simulink model "modelsim_single"  (R2016a)
settings: Solver=ode4  StartTime=0.0  StopTime=Tfinal  FixedStep=Ts  RelTol=1e-3
values from neighbouring files (symbols this model uses):
  Cdc = 100e-6    (= 0.0001)    [codemodel.m]
  delta = acos(Efm/Vt)    [codemodel.m]
  deltad = delta*180/pi    [codemodel.m]
  Ef = 155    [codemodel.m]
  fout = 50    [codemodel.m]
  Ls = 13.8e-3    (= 0.0138)    [codemodel.m]
  ma = Vt*sqrt(3)/(Vdcm*0.612)    [codemodel.m]
  phase = [0 0]    [codemodel.m]
  Rin = 10    [codemodel.m]
  Ripth = 0.08    [codemodel.m]
  Rs = 1e-9    (= 1e-09)    [codemodel.m]
  Ts = 1e-6    (= 1e-06)    [codemodel.m]
  Vin = Vdc + Rin*(Pout/Vdc)    (= 697.604412924)    [codemodel.m]
  wout = 2*pi*fout    (= 314.159265359)    [codemodel.m]
undefined symbols (not defined in the file or in its folder): Lload, Rload
libraries: powerlib x28, powerlib_meascontrol x13, simulink x2
settings Model: Creator=ugurm  LastModifiedBy=mesutto
settings DataIOCC: LimitDataPoints=on  SaveFormat=Array
settings DebuggingCC: UnderspecifiedInitializationDetection=Classic  MergeDetectMultiDrivingBlocksExec=none  SolverPrmCheckMsg=warning  StateNameClashWarn=warning
settings HardwareCC: ProdBitPerPointer=32  ProdLargestAtomicFloat=None  ProdIntDivRoundTo=Undefined  ProdEndianess=Unspecified  ProdWordSize=32  ProdHWDeviceType=32-bit Generic
settings ModelReferenceCC: PropagateSignalLabelsOutOfModel=off
settings ConfigComp: CovModelRefEnable=Off

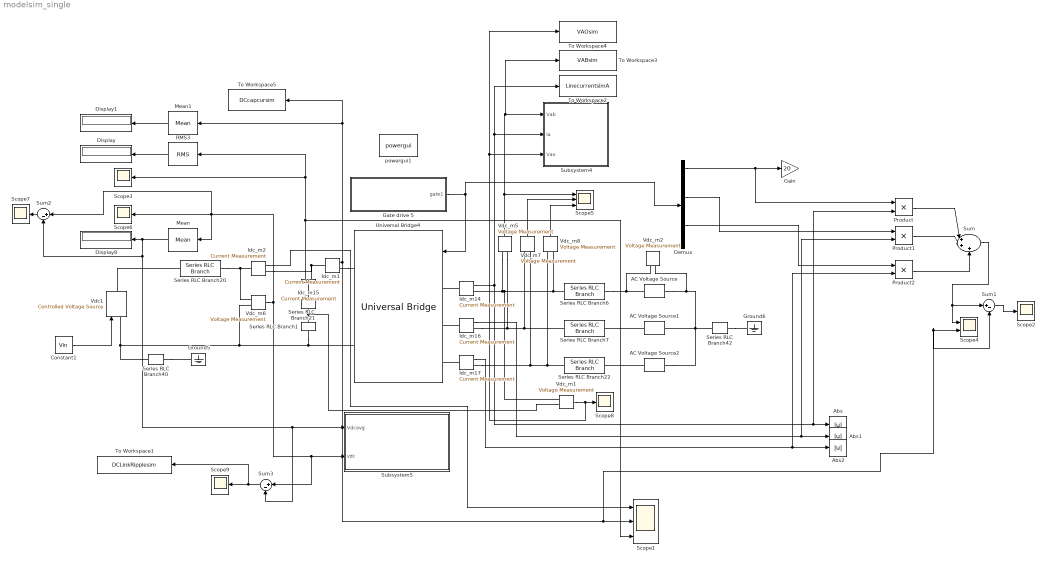
== system modelsim_single ==
  AC Voltage Source : powerlib/Electrical Sources/AC Voltage Source  Amplitude=Ef*sqrt(2)  Phase=0  Frequency=fout  SampleTime=0  Measurements=None  BusType=swing  Pref=10e3  Qref=0  Qmin=-inf  Qmax=+inf
  AC Voltage Source1 : powerlib/Electrical Sources/AC Voltage Source  Amplitude=Ef*sqrt(2)  Phase=-120  Frequency=fout  SampleTime=0  Measurements=None  BusType=swing  Pref=10e3  Qref=0  Qmin=-inf  Qmax=+inf
  AC Voltage Source2 : powerlib/Electrical Sources/AC Voltage Source  Amplitude=Ef*sqrt(2)  Phase=-240  Frequency=fout  SampleTime=0  Measurements=None  BusType=swing  Pref=10e3  Qref=0  Qmin=-inf  Qmax=+inf
  Abs : Abs
  Abs1 : Abs
  Abs2 : Abs
  Constant1 : Constant  Value=Vin
  Demux : Demux  Outputs=6
  Display : Display
  Display1 : Display
  Display8 : Display
  Gain : Gain  Gain=20
  Gate drive 5 : Subsystem
  Ground5 : powerlib/Elements/Ground  LConnTagsString=a
  Ground6 : powerlib/Elements/Ground  LConnTagsString=a
  Idc_m{1..2,14..17} (6 alike) : powerlib/Measurements/Current Measurement  PhasorSimulation=off  OutputType=Complex  PSBequivalent=0
  Mean : powerlib_meascontrol/Measurements/Mean  Freq=fout  Vinit=0  Ts=0
  Mean1 : powerlib_meascontrol/Measurements/Mean  Freq=fout  Vinit=0  Ts=0
  Product : Product
  Product1 : Product
  Product2 : Product
  RMS3 : powerlib_meascontrol/Measurements/RMS  TrueRMS=on  Freq=fout  RMSInit=0  Ts=0
  Scope1 : Scope  NumInputPorts=3
  Scope{2..3,6..9} (6 alike) : Scope
  Scope4 : Scope  NumInputPorts=2
  Scope5 : Scope  NumInputPorts=3
  Series RLC Branch1 : powerlib/Elements/Series RLC Branch  LConnTagsString=__new0  RConnTagsString=__new0  BranchType=C  Resistance=Rload  Inductance=Lload  SetiL0=off  InitialCurrent=0  Capacitance=Cdc*2  Setx0=off  InitialVoltage=0  Measurements=None
  Series RLC Branch20 : powerlib/Elements/Series RLC Branch  LConnTagsString=__new0  RConnTagsString=__new0  BranchType=R  Resistance=Rin  Inductance=Lload  SetiL0=off  InitialCurrent=0  Capacitance=1e-6  Setx0=off  InitialVoltage=0  Measurements=None
  Series RLC Branch21 : powerlib/Elements/Series RLC Branch  LConnTagsString=__new0  RConnTagsString=__new0  BranchType=C  Resistance=Rload  Inductance=Lload  SetiL0=off  InitialCurrent=0  Capacitance=Cdc*2  Setx0=off  InitialVoltage=0  Measurements=None
  Series RLC Branch22 : powerlib/Elements/Series RLC Branch  LConnTagsString=__new0  RConnTagsString=__new0  BranchType=RL  Resistance=Rs  Inductance=Ls  SetiL0=off  InitialCurrent=0  Capacitance=1e-6  Setx0=off  InitialVoltage=0  Measurements=None
  Series RLC Branch40 : powerlib/Elements/Series RLC Branch  LConnTagsString=__new0  RConnTagsString=__new0  BranchType=R  Resistance=1e12  Inductance=Lload  SetiL0=off  InitialCurrent=0  Capacitance=1e-6  Setx0=off  InitialVoltage=0  Measurements=None
  Series RLC Branch42 : powerlib/Elements/Series RLC Branch  LConnTagsString=__new0  RConnTagsString=__new0  BranchType=R  Resistance=1e12  Inductance=Lload  SetiL0=off  InitialCurrent=0  Capacitance=1e-6  Setx0=off  InitialVoltage=0  Measurements=None
  Series RLC Branch6 : powerlib/Elements/Series RLC Branch  LConnTagsString=__new0  RConnTagsString=__new0  BranchType=RL  Resistance=Rs  Inductance=Ls  SetiL0=off  InitialCurrent=0  Capacitance=1e-6  Setx0=off  InitialVoltage=0  Measurements=None
  Series RLC Branch7 : powerlib/Elements/Series RLC Branch  LConnTagsString=__new0  RConnTagsString=__new0  BranchType=RL  Resistance=Rs  Inductance=Ls  SetiL0=off  InitialCurrent=0  Capacitance=1e-6  Setx0=off  InitialVoltage=0  Measurements=None
  Subsystem4 : Subsystem
  Subsystem5 : Subsystem
  Sum : Sum  Inputs=|+++
  Sum1 : Sum  Inputs=|+-
  Sum2 : Sum  Inputs=|+-
  Sum3 : Sum  Inputs=|+-
  To Workspace1 : ToWorkspace  VariableName=DCLinkRipplesim  SampleTime=-1
  To Workspace2 : ToWorkspace  VariableName=LinecurrentsimA  SampleTime=-1
  To Workspace3 : ToWorkspace  VariableName=VABsim  SampleTime=-1
  To Workspace4 : ToWorkspace  VariableName=VAOsim  SampleTime=-1
  To Workspace5 : ToWorkspace  VariableName=DCcapcursim  SampleTime=-1
  Universal Bridge4 : powerlib/Power Electronics/Universal Bridge  Arms=3  SnubberResistance=1e5  SnubberCapacitance=inf  Device=IGBT / Diodes  Ron=1e-6  Lon=0  ForwardVoltages="[  0  0  ]"  ForwardVoltage=0  GTOparameters=[ 10e-6 , 20e-6 ]  IGBTparameters=[0,0]  Measurements=None  Measurements_2=None  converterType=Rectifier
  Vdc1 : powerlib/Electrical Sources/Controlled Voltage Source  Initialize=off  Source_Type=DC  Amplitude=200  Phase=0  Frequency=0  Measurements=None
  Vdc_m{1..2,5..8} (6 alike) : powerlib/Measurements/Voltage Measurement  PhasorSimulation=off  OutputType=Complex  PSBequivalent=0
  powergui1 : powerlib/powergui  Priority=1  SimulationMode=Discrete  SolverType=Tustin  SampleTime=Ts  frequency=60  SPID=off  DisableSnubberDevices=off  DisableRonSwitches=off  DisableVfSwitches=off  SwTol=0  DisplayEquations=off  Interpol=off  ExternalGateDelay=off  methode=off  Ts=0  FunctionMessages=off  echomessages=off  HookPort=off  EnableUseOfTLC=off  x0status=blocks  frequencyindice=0  Pbase=100e6  ErrMax=1e-4  Iterations=50  UnitsV=kV  UnitsW=MW  buscounter=0  RestoreLinks=warning  ResistiveCurrentMeasurement=off  Frange=[0:2:500]  Ylog=off  Xlog=on  ShowGrid=off  save=off  variable=ZData  structure=Vdc  ZoomFFT=off  StartTime=0.04  cycles=5  DisplayStyle=5  fundamental=50  FreqAxis=off  MaxFrequency=30000  frequencyindicesteady=1  RmsSteady=1  display=off
  wires:
  Gate drive 5/1(gate1) -> Universal Bridge4/1, Demux/1
  Vdc_m5/1 -> Scope5/1, To Workspace3/1, Subsystem4/1(Vab)
  Idc_m14/1 -> Product/2, Abs/1, To Workspace2/1, Subsystem4/2(Ia)
  Constant1/1 -> Vdc1/1
  Idc_m15/1 -> Scope1/3, RMS3/1, Scope3/1
  Vdc_m6/1 -> Sum3/1, Subsystem5/2(vdc), Sum2/1, Mean/1, Scope6/1
  Idc_m16/1 -> Product1/2, Abs1/1
  Idc_m17/1 -> Product2/2, Abs2/1
  RMS3/1 -> Display/1
  Vdc_m7/1 -> Scope5/2
  Vdc_m8/1 -> Scope5/3
  Mean/1 -> Sum2/2, Subsystem5/1(Vdcavg), Sum3/2, Display8/1
  Idc_m2/1 -> Scope1/1
  Demux/1 -> Product/1, Gain/1
  Demux/3 -> Product1/1
  Demux/5 -> Product2/1
  Product1/1 -> Sum/2
  Product/1 -> Sum/1
  Product2/1 -> Sum/3
  Sum/1 -> Sum1/1, Scope4/1
  Idc_m1/1 -> Sum1/2, Scope4/2, Scope1/2, To Workspace5/1, Mean1/1
  Sum1/1 -> Scope2/1
  Mean1/1 -> Display1/1
  Sum2/1 -> Scope7/1
  Vdc_m1/1 -> To Workspace4/1, Subsystem4/3(Vao), Scope8/1
  Sum3/1 -> To Workspace1/1, Scope9/1
  connections:
  Vdc_m5/LConn1 -- Vdc_m1/LConn1 -- Vdc_m8/LConn2 -- Series RLC Branch6/LConn1 -- Idc_m14/RConn1
  Universal Bridge4/RConn2 -- Series RLC Branch1/RConn1 -- Vdc_m6/LConn2 -- Series RLC Branch40/LConn1 -- Vdc1/LConn1
  Series RLC Branch42/RConn1 -- Ground6/LConn1
  Series RLC Branch40/RConn1 -- Ground5/LConn1
  Idc_m14/LConn1 -- Universal Bridge4/LConn1
  Idc_m15/LConn1 -- Series RLC Branch21/LConn1
  Idc_m1/LConn1 -- Idc_m2/RConn1 -- Idc_m15/RConn1
  Vdc1/RConn1 -- Series RLC Branch20/LConn1
  Series RLC Branch6/RConn1 -- Vdc_m2/LConn1 -- AC Voltage Source/RConn1
  AC Voltage Source1/RConn1 -- Series RLC Branch7/RConn1
  AC Voltage Source2/RConn1 -- Series RLC Branch22/RConn1
  Series RLC Branch42/LConn1 -- Vdc_m2/LConn2 -- AC Voltage Source/LConn1 -- AC Voltage Source2/LConn1 -- AC Voltage Source1/LConn1
  Idc_m16/LConn1 -- Universal Bridge4/LConn2
  Idc_m17/LConn1 -- Universal Bridge4/LConn3
  Idc_m17/RConn1 -- Vdc_m7/LConn2 -- Vdc_m8/LConn1 -- Series RLC Branch22/LConn1
  Idc_m16/RConn1 -- Vdc_m7/LConn1 -- Series RLC Branch7/LConn1 -- Vdc_m5/LConn2
  Idc_m1/RConn1 -- Universal Bridge4/RConn1
  Series RLC Branch20/RConn1 -- Idc_m2/LConn1 -- Vdc_m6/LConn1
  Series RLC Branch1/LConn1 -- Vdc_m1/LConn2 -- Series RLC Branch21/RConn1

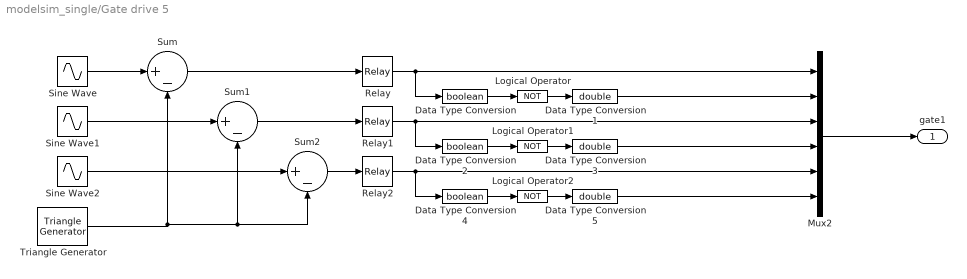
== system modelsim_single/Gate drive 5 ==
  Data Type Conversion : DataTypeConversion  OutDataTypeStr=boolean
  Data Type Conversion1 : DataTypeConversion  OutDataTypeStr=double
  Data Type Conversion2 : DataTypeConversion  OutDataTypeStr=boolean
  Data Type Conversion3 : DataTypeConversion  OutDataTypeStr=double
  Data Type Conversion4 : DataTypeConversion  OutDataTypeStr=boolean
  Data Type Conversion5 : DataTypeConversion  OutDataTypeStr=double
  Logical Operator : Logic  Operator=NOT  AllPortsSameDT=off  OutDataTypeStr=boolean
  Logical Operator1 : Logic  Operator=NOT  AllPortsSameDT=off  OutDataTypeStr=boolean
  Logical Operator2 : Logic  Operator=NOT  AllPortsSameDT=off  OutDataTypeStr=boolean
  Mux2 : Mux  Inputs=6
  Relay : Relay
  Relay1 : Relay
  Relay2 : Relay
  Sine Wave : Sin  Amplitude=ma  Frequency=wout  Phase=delta  SampleTime=0
  Sine Wave1 : Sin  Amplitude=ma  Frequency=wout  Phase=-2*pi/3+delta  SampleTime=0
  Sine Wave2 : Sin  Amplitude=ma  Frequency=wout  Phase=2*pi/3+delta  SampleTime=0
  Sum : Sum  Inputs=|+-
  Sum1 : Sum  Inputs=|+-
  Sum2 : Sum  Inputs=|+-
  Triangle Generator : powerlib_meascontrol/Pulse & Signal Generators/Triangle Generator  Freq=fsw  Phase=phase(1)  Ts=Ts
  gate1 : Outport
  wires:
  Sine Wave/1 -> Sum/1
  Triangle Generator/1 -> Sum1/2, Sum2/2, Sum/2
  Sine Wave1/1 -> Sum1/1
  Sine Wave2/1 -> Sum2/1
  Sum/1 -> Relay/1
  Sum1/1 -> Relay1/1
  Sum2/1 -> Relay2/1
  Data Type Conversion/1 -> Logical Operator/1
  Relay/1 -> Data Type Conversion/1, Mux2/1
  Logical Operator/1 -> Data Type Conversion1/1
  Data Type Conversion1/1 -> Mux2/2
  Data Type Conversion2/1 -> Logical Operator1/1
  Relay1/1 -> Data Type Conversion2/1, Mux2/3
  Logical Operator1/1 -> Data Type Conversion3/1
  Data Type Conversion3/1 -> Mux2/4
  Data Type Conversion4/1 -> Logical Operator2/1
  Relay2/1 -> Data Type Conversion4/1, Mux2/5
  Logical Operator2/1 -> Data Type Conversion5/1
  Data Type Conversion5/1 -> Mux2/6
  Mux2/1 -> gate1/1

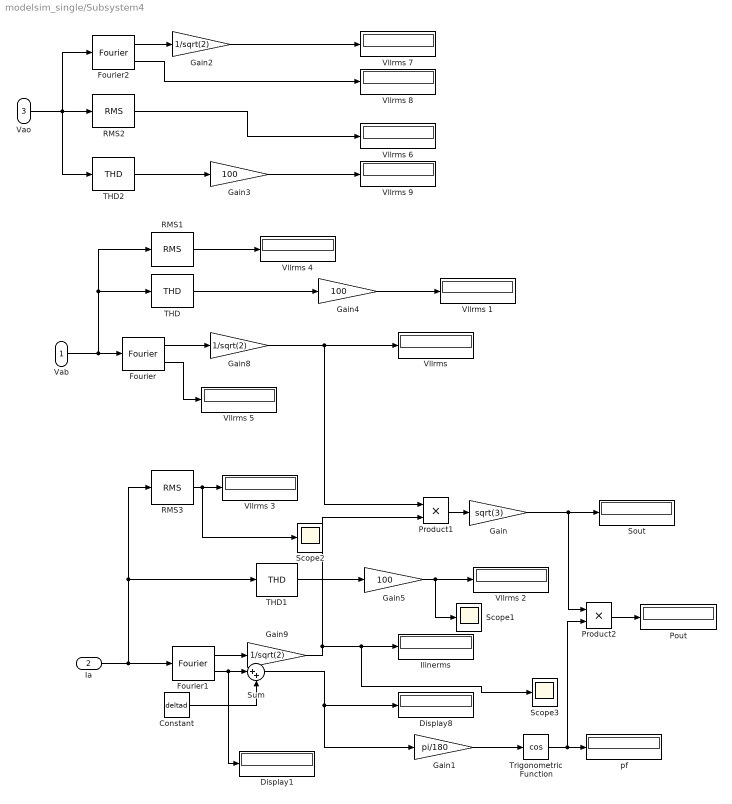
== system modelsim_single/Subsystem4 ==
  Vab : Inport
  Ia : Inport  Port=2
  Vao : Inport  Port=3
  Constant : Constant  Value=deltad
  Display1 : Display
  Display8 : Display
  Fourier : powerlib_meascontrol/Measurements/Fourier  Freq=fout  n=1  InInit=[0, 0]  Ts=Ts
  Fourier1 : powerlib_meascontrol/Measurements/Fourier  Freq=fout  n=1  InInit=[0, 0]  Ts=Ts
  Fourier2 : powerlib_meascontrol/Measurements/Fourier  Freq=fout  n=1  InInit=[0, 0]  Ts=Ts
  Gain : Gain  Gain=sqrt(3)
  Gain1 : Gain  Gain=pi/180
  Gain2 : Gain  Gain=1/sqrt(2)
  Gain3 : Gain  Gain=100
  Gain4 : Gain  Gain=100
  Gain5 : Gain  Gain=100
  Gain8 : Gain  Gain=1/sqrt(2)
  Gain9 : Gain  Gain=1/sqrt(2)
  "Ilinerms " : Display
  Pout : Display
  Product1 : Product
  Product2 : Product
  RMS1 : powerlib_meascontrol/Measurements/RMS  TrueRMS=on  Freq=fout  RMSInit=0  Ts=0
  RMS2 : powerlib_meascontrol/Measurements/RMS  TrueRMS=on  Freq=fout  RMSInit=0  Ts=0
  RMS3 : powerlib_meascontrol/Measurements/RMS  TrueRMS=on  Freq=fout  RMSInit=0  Ts=0
  Scope1 : Scope
  Scope2 : Scope
  Scope3 : Scope
  Sout : Display
      settings: Format=short_e
  Sum : Sum  Inputs=|++
  THD : powerlib_meascontrol/Measurements/THD  Freq=fout  Ts=0
  THD1 : powerlib_meascontrol/Measurements/THD  Freq=fout  Ts=0
  THD2 : powerlib_meascontrol/Measurements/THD  Freq=fout  Ts=0
  Trigonometric Function : Trigonometry  Operator=cos
  Vllrms {,1..9} (10 alike) : Display
  pf : Display
  wires:
  Gain8/1 -> Product1/1, "Vllrms "/1
  Gain9/1 -> Scope3/1, "Ilinerms "/1, Product1/2
  Ia/1 -> RMS3/1, THD1/1, Fourier1/1
  Fourier1/1 -> Gain9/1
  Vab/1 -> RMS1/1, THD/1, Fourier/1
  Fourier/1 -> Gain8/1
  Product1/1 -> Gain/1
  Gain/1 -> Product2/1, Sout/1
  Sum/1 -> Gain1/1, Display8/1
  Trigonometric Function/1 -> Product2/2, pf/1
  Gain1/1 -> Trigonometric Function/1
  Product2/1 -> Pout/1
  Fourier/2 -> Vllrms 5/1
  THD/1 -> Gain4/1
  THD1/1 -> Gain5/1
  Constant/1 -> Sum/2
  RMS3/1 -> Scope2/1, Vllrms 3/1
  RMS1/1 -> Vllrms 4/1
  Fourier1/2 -> Display1/1, Sum/1
  Vao/1 -> THD2/1, Fourier2/1, RMS2/1
  RMS2/1 -> Vllrms 6/1
  Fourier2/1 -> Gain2/1
  Fourier2/2 -> Vllrms 8/1
  Gain2/1 -> Vllrms 7/1
  THD2/1 -> Gain3/1
  Gain3/1 -> Vllrms 9/1
  Gain4/1 -> Vllrms 1/1
  Gain5/1 -> Scope1/1, Vllrms 2/1

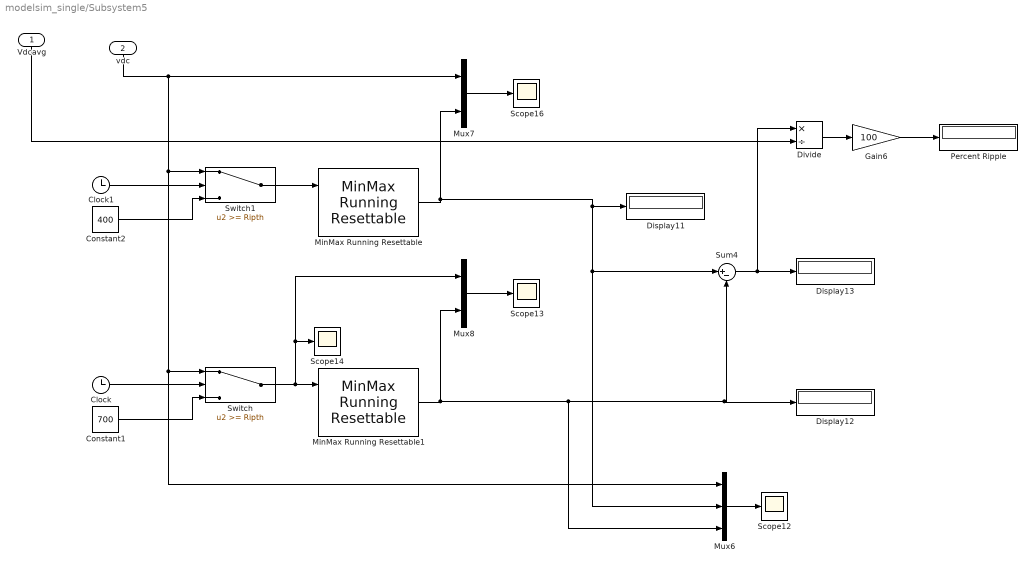
== system modelsim_single/Subsystem5 ==
  Vdcavg : Inport
  vdc : Inport  Port=2
  Clock : Clock
  Clock1 : Clock
  Constant1 : Constant  Value=700  SampleTime=Ts
  Constant2 : Constant  Value=400  SampleTime=Ts
  Display11 : Display
  Display12 : Display
  Display13 : Display
  Divide : Product  Inputs=*/
  Gain6 : Gain  Gain=100
  MinMax Running Resettable : simulink/Math Operations/MinMax Running Resettable  Function=max  vinit=0.0
  MinMax Running Resettable1 : simulink/Math Operations/MinMax Running Resettable  Function=min  vinit=700
  Mux6 : Mux  Inputs=3
  Mux7 : Mux  Inputs=2
  Mux8 : Mux  Inputs=2
  Percent Ripple : Display
  Scope{12..14,16} (4 alike) : Scope
  Sum4 : Sum  Inputs=|+-
  Switch : Switch  Threshold=Ripth
  Switch1 : Switch  Threshold=Ripth
  wires:
  MinMax Running Resettable/1 -> Display11/1, Mux6/2, Sum4/1, Mux7/2
  Clock/1 -> Switch/2
  Mux8/1 -> Scope13/1
  Gain6/1 -> Percent Ripple/1
  Constant1/1 -> Switch/3
  MinMax Running Resettable1/1 -> Mux6/3, Display12/1, Sum4/2, Mux8/2
  Mux7/1 -> Scope16/1
  Switch/1 -> Mux8/1, Scope14/1, MinMax Running Resettable1/1
  Sum4/1 -> Divide/1, Display13/1
  Divide/1 -> Gain6/1
  Mux6/1 -> Scope12/1
  Vdcavg/1 -> Divide/2
  vdc/1 -> Mux7/1, Switch1/1, Mux6/1, Switch/1
  Switch1/1 -> MinMax Running Resettable/1
  Clock1/1 -> Switch1/2
  Constant2/1 -> Switch1/3
